simulink model "regolatore_3"  (R2022b)
settings: Solver=VariableStepAuto  StartTime=0.0  StopTime=10.0  RelTol=1e-3
libraries: robotmobilelib x1, dspsigops x1
settings Model: Creator=thoma  LastModifiedBy=borgh

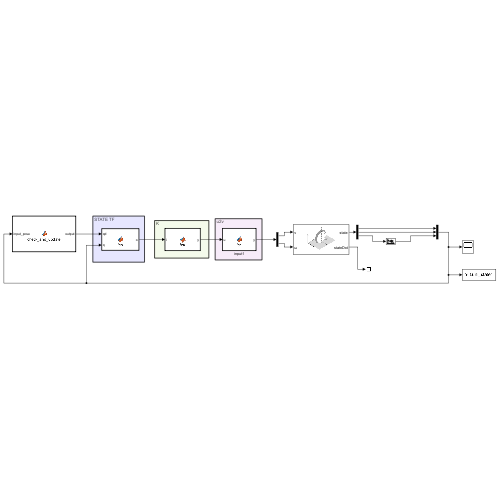
[thumbnail: Simulink's stored preview of the top-level diagram]
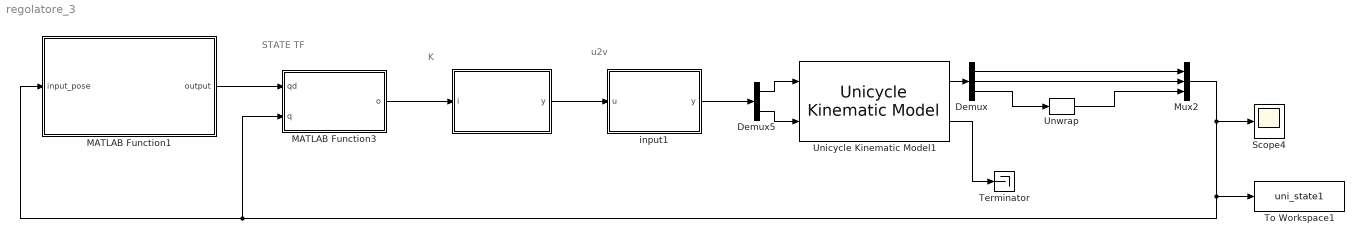
== system regolatore_3 ==
  note: u2v
  note: K
  note: STATE TF
  " " : MATLAB Function  TreatAsAtomicUnit=on
  Demux : Demux  Outputs=3
  Demux5 : Demux  Outputs=2
  MATLAB Function1 : MATLAB Function  TreatAsAtomicUnit=on
  MATLAB Function3 : MATLAB Function  TreatAsAtomicUnit=on
  Mux2 : Mux  Inputs=3
  Scope4 : Scope
  Terminator : Terminator
  To Workspace1 : ToWorkspace  VariableName=uni_state1  SaveFormat=Structure With Time  SampleTime=0.004
  Unicycle Kinematic Model1 : robotmobilelib/Unicycle Kinematic Model  VehicleInputs=Vehicle Speed & Heading Angular Velocity  WheelRadius=2  WheelSpeedRange=[-Inf Inf]  InitialState=[125;60;0]  SimulateUsing=Interpreted execution
  Unwrap : dspsigops/Unwrap  tol=pi  InputProcessing=Columns as channels (frame based)  running=off
  input1 : MATLAB Function  TreatAsAtomicUnit=on
  wires:
  Demux5/1 -> Unicycle Kinematic Model1/1
  MATLAB Function1/1(output) -> MATLAB Function3/1(qd)
  Unicycle Kinematic Model1/2 -> Terminator/1
  Demux5/2 -> Unicycle Kinematic Model1/2
  Mux2/1 -> Scope4/1, To Workspace1/1, MATLAB Function1/1(input_pose), MATLAB Function3/2(q)
  Demux/3 -> Unwrap/1
  Unicycle Kinematic Model1/1 -> Demux/1
  MATLAB Function3/1(o) -> " "/1(i)
  Demux/1 -> Mux2/1
  Unwrap/1 -> Mux2/3
  Demux/2 -> Mux2/2
  " "/1(y) -> input1/1(u)
  input1/1(y) -> Demux5/1

== matlab function regolatore_3/MATLAB Function1 ==
  settings: updateMethod=DISCRETE
  data: input_pose input; output output
function output = check_and_update(input_pose)
    % Input:
    %   input_pose - a vector [x; y; theta]
    % Output:
    %   output - a vector [x_out; y_out]

    % Define the target coordinates
   
    persistent target_y; % Define target_y as persistent so it can retain its value
    persistent has_updated; % Flag to track if the update has already occurred
    persistent target_x;
    persistent target_thet;
    % Initialize persistent variables
    if isempty(target_y)

        target_y = 60; % Initial value
        target_x=270;
        target_thet=0;
    end
    if isempty(has_updated)
        has_updated = false; % Initialize the flag
    end

    % Extract x, y from input_pose
    x = input_pose(1);
    y = input_pose(2);
    theta=input_pose(3);
    tolerance = 2;

    % Check if the pose is near the target position
    if abs(x - target_x) <= tolerance && abs(y - target_y)<= tolerance && ~has_updated  && abs(theta - target_thet) <= 0.2
        % Update y-coordinate only once

        target_y = 90;
        target_x=280;
        target_thet=pi/2;
        has_updated = true; % Set the flag to prevent future updates
    end

    % Output the updated or unchanged target coordinates
    output = [target_x; target_y;target_thet];
end

== matlab function regolatore_3/MATLAB Function3 ==
  data: qd input; o output; q input
function o = fcn(qd,q)
    xi=q(1);
    yi=q(2);
    thetai=q(3);

    R = [cos(qd(3)), sin(qd(3));
        -sin(qd(3)), cos(qd(3))];
    

    x = (xi - qd(1));
    y = (yi - qd(2));
    theta = (thetai - qd(3));

    xy_new = (R * [x; y])';
    x = xy_new(1);
    y = xy_new(2);


    theta=mod(theta+pi,2*pi)-pi;

    rho=sqrt(x^2+y^2);
    gamma=atan2(y,x)+pi-theta;
    delta=gamma+theta;

    delta=mod(delta+pi,2*pi)-pi;
    gamma=mod(gamma+pi,2*pi)-pi;

    o = [rho;gamma;delta];

== matlab function regolatore_3/input1 ==
  data: u input; y output
function y = fcn(u)
    v=u(2)*u(1);
    w=u(3);

    y = [v;w];

== matlab function regolatore_3/  ==
  data: i input; y output
function y = fcn(i)
    k1=10;
    k2=40;
    k3=8;
    
    rho=i(1);
    gamma=i(2);
    delta=i(3);

    u=k1*cos(gamma);
    
    if gamma > 0.0001
        w = k2 * gamma + k1 * sin(gamma) * cos(gamma) / gamma * (gamma + k3 * delta);
    else
        w=0;
    end

    y = [rho;u;w];
